simulink model "taskBasedBalancing"  (Simulink 9.0)
settings: Solver=FixedStepDiscrete  StartTime=0.0  StopTime=Config.t_end  FixedStep=Config.t_step  RelTol=1e-3  EnableMultiTasking=on
InitFcn:
  | cd(fileparts(which(bdroot)));
  | initTaskBasedBalancing;
StopFcn:
  | cd(fileparts(which(bdroot)));
  | stopTaskBasedBalancing;
undefined symbols (not defined in the file or in its folder): Config, DiscIntNeverNeededParam, Gains, ROBOT_DOF, Sat
libraries: WBToolboxLibrary x66
(part 2 of 2)

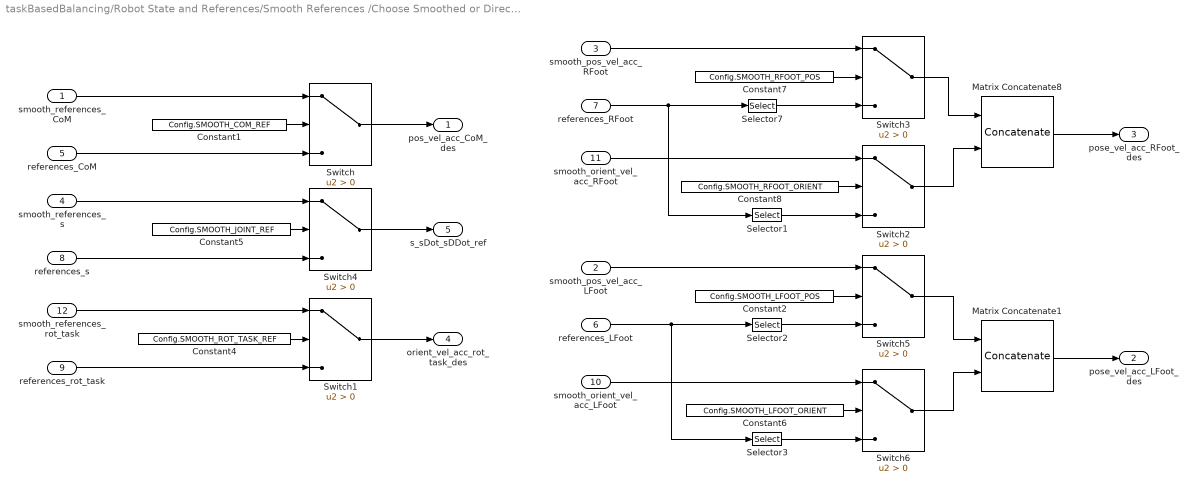
== system taskBasedBalancing/Robot State and References/Smooth References /Choose Smoothed or Direct References ==
  smooth_references_CoM : Inport
  smooth_pos_vel_acc_LFoot : Inport  Port=2
  smooth_pos_vel_acc_RFoot : Inport  Port=3
  smooth_references_s : Inport  Port=4
  references_CoM : Inport  Port=5
  references_LFoot : Inport  Port=6
  references_RFoot : Inport  Port=7
  references_s : Inport  Port=8
  references_rot_task : Inport  Port=9
  smooth_orient_vel_acc_LFoot : Inport  Port=10
  smooth_orient_vel_acc_RFoot : Inport  Port=11
  smooth_references_rot_task : Inport  Port=12
  Constant1 : Constant  Value=Config.SMOOTH_COM_REF
  Constant2 : Constant  Value=Config.SMOOTH_LFOOT_POS
  Constant4 : Constant  Value=Config.SMOOTH_ROT_TASK_REF
  Constant5 : Constant  Value=Config.SMOOTH_JOINT_REF
  Constant6 : Constant  Value=Config.SMOOTH_LFOOT_ORIENT
  Constant7 : Constant  Value=Config.SMOOTH_RFOOT_POS
  Constant8 : Constant  Value=Config.SMOOTH_RFOOT_ORIENT
  Matrix Concatenate1 : Concatenate  Mode=Multidimensional array
  Matrix Concatenate8 : Concatenate  Mode=Multidimensional array
  Selector1 : Selector  NumberOfDimensions=2  InputPortWidth=ROBOT_DOF  IndexOptions=Index vector (dialog),Index vector (dialog)  Indices=[4:6],[1:5]  OutputSizes=1,1
  Selector2 : Selector  NumberOfDimensions=2  InputPortWidth=ROBOT_DOF  IndexOptions=Index vector (dialog),Index vector (dialog)  Indices=[1:3],[1:5]  OutputSizes=1,1
  Selector3 : Selector  NumberOfDimensions=2  InputPortWidth=ROBOT_DOF  IndexOptions=Index vector (dialog),Index vector (dialog)  Indices=[4:6],[1:5]  OutputSizes=1,1
  Selector7 : Selector  NumberOfDimensions=2  InputPortWidth=ROBOT_DOF  IndexOptions=Index vector (dialog),Index vector (dialog)  Indices=[1:3],[1:5]  OutputSizes=1,1
  Switch{,1..6} (7 alike) : Switch  Criteria=u2 > Threshold
  pos_vel_acc_CoM_des : Outport
  pose_vel_acc_LFoot_des : Outport  Port=2
  pose_vel_acc_RFoot_des : Outport  Port=3
  orient_vel_acc_rot_task_des : Outport  Port=4
  s_sDot_sDDot_ref : Outport  Port=5
  wires:
  Constant1/1 -> Switch/2
  Switch/1 -> pos_vel_acc_CoM_des/1
  Constant5/1 -> Switch4/2
  Switch4/1 -> s_sDot_sDDot_ref/1
  references_CoM/1 -> Switch/3
  smooth_references_CoM/1 -> Switch/1
  smooth_references_s/1 -> Switch4/1
  references_s/1 -> Switch4/3
  smooth_references_rot_task/1 -> Switch1/1
  references_rot_task/1 -> Switch1/3
  Constant4/1 -> Switch1/2
  Switch1/1 -> orient_vel_acc_rot_task_des/1
  smooth_pos_vel_acc_RFoot/1 -> Switch3/1
  Constant7/1 -> Switch3/2
  references_RFoot/1 -> Selector1/1, Selector7/1
  Selector7/1 -> Switch3/3
  smooth_orient_vel_acc_RFoot/1 -> Switch2/1
  Constant8/1 -> Switch2/2
  Selector1/1 -> Switch2/3
  Switch3/1 -> Matrix Concatenate8/1
  Switch2/1 -> Matrix Concatenate8/2
  references_LFoot/1 -> Selector3/1, Selector2/1
  Matrix Concatenate8/1 -> pose_vel_acc_RFoot_des/1
  Constant6/1 -> Switch6/2
  Matrix Concatenate1/1 -> pose_vel_acc_LFoot_des/1
  Switch5/1 -> Matrix Concatenate1/1
  Switch6/1 -> Matrix Concatenate1/2
  Constant2/1 -> Switch5/2
  Selector2/1 -> Switch5/3
  smooth_pos_vel_acc_LFoot/1 -> Switch5/1
  smooth_orient_vel_acc_LFoot/1 -> Switch6/1
  Selector3/1 -> Switch6/3

== system taskBasedBalancing/Robot State and References/Smooth References /Smooth Reference Orientations ==
  w_R_LFoot_des : Inport
  w_R_RFoot_des : Inport  Port=2
  w_R_Rot_task_des : Inport  Port=3
  state : Inport  Port=4
  Compose Smoothed References : Subsystem
  Compute Smoothed Ref Orientations : Subsystem
  Constant{,1..5} (6 alike) : Constant  Value=zeros(3,1)
  smooth_orient_vel_acc_LFoot : Outport
  smooth_orient_vel_acc_RFoot : Outport  Port=2
  smooth_orient_vel_acc_Rot_task : Outport  Port=3
  wires:
  w_R_LFoot_des/1 -> Compute Smoothed Ref Orientations/1(w_R_LFoot_des)
  w_R_RFoot_des/1 -> Compute Smoothed Ref Orientations/2(w_R_RFoot_des)
  w_R_Rot_task_des/1 -> Compute Smoothed Ref Orientations/3(w_R_rot_task_des)
  Compute Smoothed Ref Orientations/3(w_R_LFoot) -> Compose Smoothed References/6(w_R_LFoot)
  Compute Smoothed Ref Orientations/2(w_R_RFoot) -> Compose Smoothed References/5(w_R_RFoot)
  Compute Smoothed Ref Orientations/1(w_R_rot_task) -> Compose Smoothed References/4(w_R_rot_task)
  Compose Smoothed References/1(orient_vel_acc_LFoot_des) -> smooth_orient_vel_acc_LFoot/1
  Compose Smoothed References/2(orient_vel_acc_RFoot_des) -> smooth_orient_vel_acc_RFoot/1
  Compose Smoothed References/3(orient_vel_acc_rot_task_des) -> smooth_orient_vel_acc_Rot_task/1
  state/1 -> Compute Smoothed Ref Orientations/4(state)
  Constant/1 -> Compose Smoothed References/1(omegaDot_LFoot)
  Constant1/1 -> Compose Smoothed References/2(omegaDot_RFoot)
  Constant2/1 -> Compose Smoothed References/3(omegaDot_rot_task)
  Constant5/1 -> Compose Smoothed References/9(omega_rot_task)
  Constant4/1 -> Compose Smoothed References/8(omega_RFoot)
  Constant3/1 -> Compose Smoothed References/7(omega_LFoot)

== system taskBasedBalancing/Robot State and References/Smooth References /Smooth Reference Positions ==
  pos_CoM_des : Inport
  pos_LFoot_des : Inport  Port=2
  pos_RFoot_des : Inport  Port=3
  s_des : Inport  Port=4
  state : Inport  Port=5
  Configure Settling Times : MATLAB Function  TreatAsAtomicUnit=on
  Matrix Concatenate1 : Concatenate  NumInputs=3  Mode=Multidimensional array  ConcatenateDimension=2
  Matrix Concatenate2 : Concatenate  NumInputs=4  Mode=Multidimensional array  ConcatenateDimension=2
  Matrix Concatenate3 : Concatenate  NumInputs=4  Mode=Multidimensional array  ConcatenateDimension=2
  Matrix Concatenate4 : Concatenate  NumInputs=3  Mode=Multidimensional array  ConcatenateDimension=2
  Minimum Jerk Trajectory Generator{,1..3} (4 alike) : WBToolboxLibrary/Utilities/Minimum Jerk Trajectory Generator  externalSettlingTime=on  settlingTime=3  sampleTime=Config.t_step  resetOnSettlingTime=off  firstDerivatives=on  secondDerivatives=on  explicitInitialValue=off
      settings: SourceProductName=Whole Body Toolbox
  Settling time1 : Constant  Value=zeros(3,2)
  smooth_references_CoM : Outport
  smooth_pos_vel_acc_LFoot : Outport  Port=2
  smooth_pos_vel_acc_RFoot : Outport  Port=3
  smooth_references_s : Outport  Port=4
  wires:
  Minimum Jerk Trajectory Generator2/2 -> Matrix Concatenate3/2
  pos_LFoot_des/1 -> Minimum Jerk Trajectory Generator2/1
  pos_RFoot_des/1 -> Minimum Jerk Trajectory Generator3/1
  Minimum Jerk Trajectory Generator2/3 -> Matrix Concatenate3/3
  Minimum Jerk Trajectory Generator2/1 -> Matrix Concatenate3/1
  Minimum Jerk Trajectory Generator1/3 -> Matrix Concatenate1/3
  Matrix Concatenate1/1 -> smooth_references_s/1
  Matrix Concatenate4/1 -> smooth_references_CoM/1
  Minimum Jerk Trajectory Generator1/1 -> Matrix Concatenate1/1
  pos_CoM_des/1 -> Minimum Jerk Trajectory Generator/1
  Minimum Jerk Trajectory Generator/3 -> Matrix Concatenate4/3
  Minimum Jerk Trajectory Generator/2 -> Matrix Concatenate4/2
  Minimum Jerk Trajectory Generator1/2 -> Matrix Concatenate1/2
  Minimum Jerk Trajectory Generator3/3 -> Matrix Concatenate2/3
  Matrix Concatenate3/1 -> smooth_pos_vel_acc_LFoot/1
  Matrix Concatenate2/1 -> smooth_pos_vel_acc_RFoot/1
  Minimum Jerk Trajectory Generator/1 -> Matrix Concatenate4/1
  Minimum Jerk Trajectory Generator3/2 -> Matrix Concatenate2/2
  s_des/1 -> Minimum Jerk Trajectory Generator1/1
  Settling time1/1 -> Matrix Concatenate2/4, Matrix Concatenate3/4
  Minimum Jerk Trajectory Generator3/1 -> Matrix Concatenate2/1
  state/1 -> Configure Settling Times/1(state)
  Configure Settling Times/1(smoothingTime_CoM) -> Minimum Jerk Trajectory Generator/2
  Configure Settling Times/2(smoothingTime_joints) -> Minimum Jerk Trajectory Generator1/2
  Configure Settling Times/3(smoothingTime_LFoot) -> Minimum Jerk Trajectory Generator2/2
  Configure Settling Times/4(smoothingTime_RFoot) -> Minimum Jerk Trajectory Generator3/2

== system taskBasedBalancing/Robot State and References/State Machine/Compute Transformation Matrices ==
  s : Inport
  IMU port : Inport  Port=2
  Constant : Constant  Value=Config.LEFT_FOOT_IN_CONTACT
  Constant6 : Constant  Value=eye(4)
  "Inv\\*  " : Product  Inputs=/  Multiplication=Matrix(*)
  LFoot to base link transform : Subsystem
  LFoot to world transform (fixed base) : WBToolboxLibrary/wholeBodyModel/Kinematics/Forward Kinematics  frameName=Frames.LEFT_FOOT
      settings: SourceProductName=Whole Body Toolbox
  RFoot to base link transform : Subsystem
  RFoot to world transform (fixed base) : WBToolboxLibrary/wholeBodyModel/Kinematics/Forward Kinematics  frameName=Frames.RIGHT_FOOT
      settings: SourceProductName=Whole Body Toolbox
  Switch : Switch  Criteria=u2 > Threshold
  w_H_b_initial : Outport
  b_H_LFoot : Outport  Port=2
  b_H_RFoot : Outport  Port=3
  wires:
  s/1 -> RFoot to world transform (fixed base)/2, LFoot to world transform (fixed base)/2, RFoot to base link transform/1(s), LFoot to base link transform/1(s)
  RFoot to base link transform/1(b_H_link_corrected) -> Switch/3, b_H_RFoot/1
  LFoot to world transform (fixed base)/1 -> LFoot to base link transform/3(b_H_link)
  IMU port/1 -> RFoot to base link transform/2(inertial), LFoot to base link transform/2(inertial)
  Constant6/1 -> LFoot to world transform (fixed base)/1, RFoot to world transform (fixed base)/1
  RFoot to world transform (fixed base)/1 -> RFoot to base link transform/3(b_H_link)
  LFoot to base link transform/1(b_H_link_corrected) -> Switch/1, b_H_LFoot/1
  Switch/1 -> "Inv\\*  "/1
  Constant/1 -> Switch/2
  "Inv\\*  "/1 -> w_H_b_initial/1

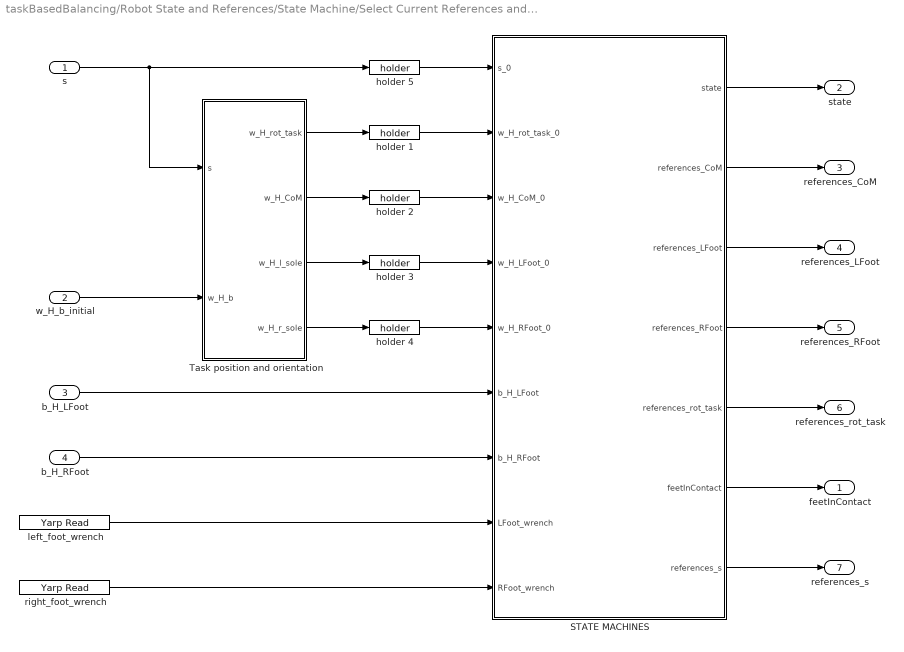
== system taskBasedBalancing/Robot State and References/State Machine/Select Current References and Estimate w_H_b ==
  s : Inport
  w_H_b_initial : Inport  Port=2
  b_H_LFoot : Inport  Port=3
  b_H_RFoot : Inport  Port=4
  STATE MACHINES : MATLAB Function  TreatAsAtomicUnit=on
  Task position and orientation : Subsystem
  holder {1..5} (5 alike) : WBToolboxLibrary/Utilities/holder 
      settings: SourceProductName=Whole Body Toolbox
  left_foot_wrench : WBToolboxLibrary/Utilities/Yarp Read  portName=Ports.LEFT_FOOT_EXT_WRENCH  signalSize=6  timeout=0.5  blocking=off  timestamp=off  autoconnect=on  errorOnConnection=on
      settings: SourceProductName=Whole Body Toolbox
  right_foot_wrench : WBToolboxLibrary/Utilities/Yarp Read  portName=Ports.RIGHT_FOOT_EXT_WRENCH  signalSize=6  timeout=0.5  blocking=off  timestamp=off  autoconnect=on  errorOnConnection=on
      settings: SourceProductName=Whole Body Toolbox
  feetInContact : Outport
  state : Outport  Port=2
  references_CoM : Outport  Port=3
  references_LFoot : Outport  Port=4
  references_RFoot : Outport  Port=5
  references_rot_task : Outport  Port=6
  references_s : Outport  Port=7
  wires:
  s/1 -> Task position and orientation/1(s), holder 5/1
  w_H_b_initial/1 -> Task position and orientation/2(w_H_b)
  holder 5/1 -> STATE MACHINES/1(s_0)
  Task position and orientation/1(w_H_rot_task) -> holder 1/1
  holder 1/1 -> STATE MACHINES/2(w_H_rot_task_0)
  b_H_RFoot/1 -> STATE MACHINES/7(b_H_RFoot)
  b_H_LFoot/1 -> STATE MACHINES/6(b_H_LFoot)
  left_foot_wrench/1 -> STATE MACHINES/8(LFoot_wrench)
  right_foot_wrench/1 -> STATE MACHINES/9(RFoot_wrench)
  STATE MACHINES/1(state) -> state/1
  STATE MACHINES/2(references_CoM) -> references_CoM/1
  STATE MACHINES/3(references_LFoot) -> references_LFoot/1
  STATE MACHINES/4(references_RFoot) -> references_RFoot/1
  STATE MACHINES/5(references_rot_task) -> references_rot_task/1
  STATE MACHINES/6(feetInContact) -> feetInContact/1
  STATE MACHINES/7(references_s) -> references_s/1
  Task position and orientation/4(w_H_r_sole) -> holder 4/1
  Task position and orientation/3(w_H_l_sole) -> holder 3/1
  Task position and orientation/2(w_H_CoM) -> holder 2/1
  holder 4/1 -> STATE MACHINES/5(w_H_RFoot_0)
  holder 3/1 -> STATE MACHINES/4(w_H_LFoot_0)
  holder 2/1 -> STATE MACHINES/3(w_H_CoM_0)

== system taskBasedBalancing/Robot State and References/State Machine/emergency stop: joint limits ==
  s   EMERGENCY STOP : Inport
  Enable : EnablePort
  Assertion : Assertion
  Get Limits : WBToolboxLibrary/wholeBodyStates/Get Limits  limitsSource=ControlBoard  limitsType=Position
      settings: SourceProductName=Whole Body Toolbox
  MATLAB Function : MATLAB Function  TreatAsAtomicUnit=on
  index1 : Constant  Value=0.01  VectorParams1D=off
  wires:
  Get Limits/1 -> MATLAB Function/1(umin)
  Get Limits/2 -> MATLAB Function/2(umax)
  index1/1 -> MATLAB Function/4(tol)
  s   EMERGENCY STOP/1 -> MATLAB Function/3(u)
  MATLAB Function/1(inRange) -> Assertion/1

== system taskBasedBalancing/Visualization/Visualize Smoothing (orientation)/Rotation Error Left Foot ==
  w_R_LFoot : Inport
  w_R_LFoot_des : Inport  Port=2
  Permute Dimensions2 : PermuteDimensions
  Product2 : Product  Multiplication=Matrix(*)
  Rot error using roll-pitch-yaw : MATLAB Function  TreatAsAtomicUnit=on
  rollPitchYaw : Outport
  wires:
  w_R_LFoot_des/1 -> Product2/2
  w_R_LFoot/1 -> Permute Dimensions2/1
  Permute Dimensions2/1 -> Product2/1
  Rot error using roll-pitch-yaw/1(rollPitchYaw) -> rollPitchYaw/1
  Product2/1 -> Rot error using roll-pitch-yaw/1(R_0)

== system taskBasedBalancing/Visualization/Visualize Smoothing (orientation)/Rotation Error Right Foot ==
  w_R_RFoot : Inport
  w_R_RFoot_des : Inport  Port=2
  Permute Dimensions2 : PermuteDimensions
  Product2 : Product  Multiplication=Matrix(*)
  Rot error using roll-pitch-yaw : MATLAB Function  TreatAsAtomicUnit=on
  rollPitchYaw : Outport
  wires:
  w_R_RFoot_des/1 -> Product2/2
  w_R_RFoot/1 -> Permute Dimensions2/1
  Permute Dimensions2/1 -> Product2/1
  Rot error using roll-pitch-yaw/1(rollPitchYaw) -> rollPitchYaw/1
  Product2/1 -> Rot error using roll-pitch-yaw/1(R_0)

== system taskBasedBalancing/Visualization/Visualize Smoothing (orientation)/Rotation Error Rot Task ==
  w_R_rot_task : Inport
  w_R_rot_task_des : Inport  Port=2
  Permute Dimensions2 : PermuteDimensions
  Product2 : Product  Multiplication=Matrix(*)
  Rot error using roll-pitch-yaw : MATLAB Function  TreatAsAtomicUnit=on
  rollPitchYaw : Outport
  wires:
  w_R_rot_task_des/1 -> Product2/2
  w_R_rot_task/1 -> Permute Dimensions2/1
  Permute Dimensions2/1 -> Product2/1
  Rot error using roll-pitch-yaw/1(rollPitchYaw) -> rollPitchYaw/1
  Product2/1 -> Rot error using roll-pitch-yaw/1(R_0)

== system taskBasedBalancing/Robot State and References/Smooth References /Smooth Reference Orientations/Compose Smoothed References ==
  omegaDot_LFoot : Inport
  omegaDot_RFoot : Inport  Port=2
  omegaDot_rot_task : Inport  Port=3
  w_R_rot_task : Inport  Port=4
  w_R_RFoot : Inport  Port=5
  w_R_LFoot : Inport  Port=6
  omega_LFoot : Inport  Port=7
  omega_RFoot : Inport  Port=8
  omega_rot_task : Inport  Port=9
  Matrix Concatenate1 : Concatenate  NumInputs=3  Mode=Multidimensional array  ConcatenateDimension=2
  Matrix Concatenate2 : Concatenate  NumInputs=3  Mode=Multidimensional array  ConcatenateDimension=2
  Matrix Concatenate6 : Concatenate  NumInputs=3  Mode=Multidimensional array  ConcatenateDimension=2
  orient_vel_acc_LFoot_des : Outport
  orient_vel_acc_RFoot_des : Outport  Port=2
  orient_vel_acc_rot_task_des : Outport  Port=3
  wires:
  w_R_LFoot/1 -> Matrix Concatenate6/1
  Matrix Concatenate6/1 -> orient_vel_acc_LFoot_des/1
  Matrix Concatenate2/1 -> orient_vel_acc_rot_task_des/1
  Matrix Concatenate1/1 -> orient_vel_acc_RFoot_des/1
  omega_LFoot/1 -> Matrix Concatenate6/2
  omega_RFoot/1 -> Matrix Concatenate1/2
  w_R_RFoot/1 -> Matrix Concatenate1/1
  omega_rot_task/1 -> Matrix Concatenate2/2
  w_R_rot_task/1 -> Matrix Concatenate2/1
  omegaDot_LFoot/1 -> Matrix Concatenate6/3
  omegaDot_RFoot/1 -> Matrix Concatenate1/3
  omegaDot_rot_task/1 -> Matrix Concatenate2/3

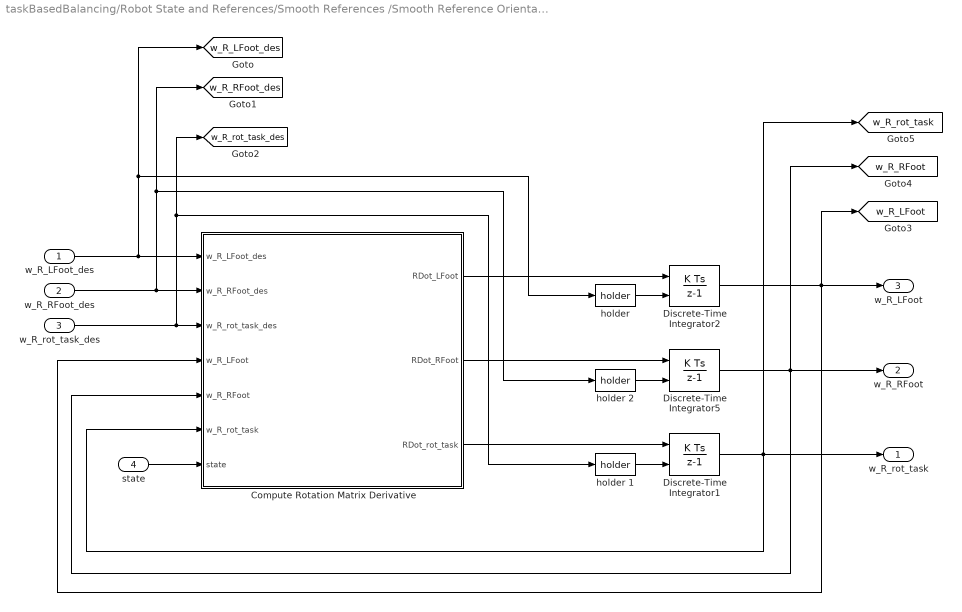
== system taskBasedBalancing/Robot State and References/Smooth References /Smooth Reference Orientations/Compute Smoothed Ref Orientations ==
  w_R_LFoot_des : Inport
  w_R_RFoot_des : Inport  Port=2
  w_R_rot_task_des : Inport  Port=3
  state : Inport  Port=4
  Compute Rotation Matrix Derivative : MATLAB Function  TreatAsAtomicUnit=on
  Discrete-Time Integrator1 : DiscreteIntegrator  InitialConditionSource=external  InitialCondition=zeros(3,1)  InitialConditionSetting=State (most efficient)  SampleTime=Config.t_step  ICPrevOutput=DiscIntNeverNeededParam  ICPrevScaledInput=DiscIntNeverNeededParam
  Discrete-Time Integrator2 : DiscreteIntegrator  InitialConditionSource=external  InitialCondition=zeros(3,1)  InitialConditionSetting=State (most efficient)  SampleTime=Config.t_step  ICPrevOutput=DiscIntNeverNeededParam  ICPrevScaledInput=DiscIntNeverNeededParam
  Discrete-Time Integrator5 : DiscreteIntegrator  InitialConditionSource=external  InitialCondition=zeros(3,1)  InitialConditionSetting=State (most efficient)  SampleTime=Config.t_step  ICPrevOutput=DiscIntNeverNeededParam  ICPrevScaledInput=DiscIntNeverNeededParam
  "holder " : WBToolboxLibrary/Utilities/holder 
      settings: SourceProductName=Whole Body Toolbox
  holder 1 : WBToolboxLibrary/Utilities/holder 
      settings: SourceProductName=Whole Body Toolbox
  holder 2 : WBToolboxLibrary/Utilities/holder 
      settings: SourceProductName=Whole Body Toolbox
  w_R_rot_task : Outport
  w_R_RFoot : Outport  Port=2
  w_R_LFoot : Outport  Port=3
  tag scope: w_R_LFoot=global, w_R_LFoot_des=global, w_R_RFoot=global, w_R_RFoot_des=global, w_R_rot_task=global, w_R_rot_task_des=global
  wires:
  "holder "/1 -> Discrete-Time Integrator2/2
  holder 2/1 -> Discrete-Time Integrator5/2
  holder 1/1 -> Discrete-Time Integrator1/2
  Compute Rotation Matrix Derivative/1(RDot_LFoot) -> Discrete-Time Integrator2/1
  Compute Rotation Matrix Derivative/2(RDot_RFoot) -> Discrete-Time Integrator5/1
  Compute Rotation Matrix Derivative/3(RDot_rot_task) -> Discrete-Time Integrator1/1
  Discrete-Time Integrator5/1 -> w_R_RFoot/1, [w_R_RFoot], Compute Rotation Matrix Derivative/5(w_R_RFoot)
  Discrete-Time Integrator1/1 -> [w_R_rot_task], w_R_rot_task/1, Compute Rotation Matrix Derivative/6(w_R_rot_task)
  Discrete-Time Integrator2/1 -> [w_R_LFoot], w_R_LFoot/1, Compute Rotation Matrix Derivative/4(w_R_LFoot)
  w_R_LFoot_des/1 -> Compute Rotation Matrix Derivative/1(w_R_LFoot_des), [w_R_LFoot_des], "holder "/1
  w_R_RFoot_des/1 -> Compute Rotation Matrix Derivative/2(w_R_RFoot_des), [w_R_RFoot_des], holder 2/1
  w_R_rot_task_des/1 -> Compute Rotation Matrix Derivative/3(w_R_rot_task_des), holder 1/1, [w_R_rot_task_des]
  state/1 -> Compute Rotation Matrix Derivative/7(state)

== system taskBasedBalancing/Robot State and References/State Machine/Compute Transformation Matrices/LFoot to base link transform ==
  s : Inport
  inertial : Inport  Port=2
  b_H_link : Inport  Port=3
  Constant6 : Constant  Value=eye(4)
  Fixed base to imu transform : WBToolboxLibrary/wholeBodyModel/Kinematics/Forward Kinematics  frameName=Frames.IMU
      settings: SourceProductName=Whole Body Toolbox
  Inv\* : Product  Inputs=/*  Multiplication=Matrix(*)
  "Inv\\*  " : Product  Inputs=/  Multiplication=Matrix(*)
  Inv\*  1 : Product  Inputs=/  Multiplication=Matrix(*)
  Neck Position : WBToolboxLibrary/Utilities/Yarp Read  portName=Ports.NECK_POS  signalSize=6  timeout=0.5  blocking=off  timestamp=off  autoconnect=on  errorOnConnection=off
      settings: SourceProductName=Whole Body Toolbox
  Switch6 : Switch  Criteria=u2 > Threshold
  USE_IMU4EST_BASE : Constant  Value=Config.USE_IMU4EST_BASE
  fromImuToHomogeousTransformFCN : MATLAB Function  TreatAsAtomicUnit=on
  holder 1 : WBToolboxLibrary/Utilities/holder 
      settings: SourceProductName=Whole Body Toolbox
  holder 2 : WBToolboxLibrary/Utilities/holder 
      settings: SourceProductName=Whole Body Toolbox
  neck transform : Subsystem
  b_H_link_corrected : Outport
  wires:
  Switch6/1 -> b_H_link_corrected/1
  "Inv\\*  "/1 -> fromImuToHomogeousTransformFCN/3(link_H_base)  "link_H_b"
  USE_IMU4EST_BASE/1 -> Switch6/2
  Inv\*/1 -> fromImuToHomogeousTransformFCN/1(imu_H_link), holder 1/1  "imu_H_link"
  holder 2/1 -> fromImuToHomogeousTransformFCN/4(inertial_0)
  Fixed base to imu transform/1 -> Inv\*/1
  holder 1/1 -> fromImuToHomogeousTransformFCN/2(imu_H_link_0)
  s/1 -> Fixed base to imu transform/2
  fromImuToHomogeousTransformFCN/1(w_H_b) -> Inv\*  1/1
  inertial/1 -> holder 2/1, fromImuToHomogeousTransformFCN/5(inertial)
  Neck Position/1 -> neck transform/1(neck port)
  neck transform/1(neck position) -> fromImuToHomogeousTransformFCN/6(neck_pos)
  b_H_link/1 -> Switch6/3, "Inv\\*  "/1, Inv\*/2
  Constant6/1 -> Fixed base to imu transform/1
  Inv\*  1/1 -> Switch6/1

== system taskBasedBalancing/Robot State and References/State Machine/Compute Transformation Matrices/RFoot to base link transform ==
  s : Inport
  inertial : Inport  Port=2
  b_H_link : Inport  Port=3
  Constant6 : Constant  Value=eye(4)
  Fixed base to imu transform : WBToolboxLibrary/wholeBodyModel/Kinematics/Forward Kinematics  frameName=Frames.IMU
      settings: SourceProductName=Whole Body Toolbox
  Inv\* : Product  Inputs=/*  Multiplication=Matrix(*)
  "Inv\\*  " : Product  Inputs=/  Multiplication=Matrix(*)
  Inv\*  1 : Product  Inputs=/  Multiplication=Matrix(*)
  Neck Position : WBToolboxLibrary/Utilities/Yarp Read  portName=Ports.NECK_POS  signalSize=6  timeout=0.5  blocking=off  timestamp=off  autoconnect=on  errorOnConnection=off
      settings: SourceProductName=Whole Body Toolbox
  Switch6 : Switch  Criteria=u2 > Threshold
  USE_IMU4EST_BASE : Constant  Value=Config.USE_IMU4EST_BASE
  fromImuToHomogeousTransformFCN : MATLAB Function  TreatAsAtomicUnit=on
  holder 1 : WBToolboxLibrary/Utilities/holder 
      settings: SourceProductName=Whole Body Toolbox
  holder 2 : WBToolboxLibrary/Utilities/holder 
      settings: SourceProductName=Whole Body Toolbox
  neck transform : Subsystem
  b_H_link_corrected : Outport
  wires:
  Switch6/1 -> b_H_link_corrected/1
  "Inv\\*  "/1 -> fromImuToHomogeousTransformFCN/3(link_H_base)  "link_H_b"
  USE_IMU4EST_BASE/1 -> Switch6/2
  Inv\*/1 -> fromImuToHomogeousTransformFCN/1(imu_H_link), holder 1/1  "imu_H_link"
  holder 2/1 -> fromImuToHomogeousTransformFCN/4(inertial_0)
  Fixed base to imu transform/1 -> Inv\*/1
  holder 1/1 -> fromImuToHomogeousTransformFCN/2(imu_H_link_0)
  s/1 -> Fixed base to imu transform/2
  fromImuToHomogeousTransformFCN/1(w_H_b) -> Inv\*  1/1
  inertial/1 -> holder 2/1, fromImuToHomogeousTransformFCN/5(inertial)
  Neck Position/1 -> neck transform/1(neck port)
  neck transform/1(neck position) -> fromImuToHomogeousTransformFCN/6(neck_pos)
  b_H_link/1 -> Switch6/3, "Inv\\*  "/1, Inv\*/2
  Constant6/1 -> Fixed base to imu transform/1
  Inv\*  1/1 -> Switch6/1

== system taskBasedBalancing/Robot State and References/State Machine/Select Current References and Estimate w_H_b/Task position and orientation ==
  s : Inport
  w_H_b : Inport  Port=2
  CoM : WBToolboxLibrary/wholeBodyModel/Kinematics/Forward Kinematics  frameName=Frames.COM
      settings: SourceProductName=Whole Body Toolbox
  LFoot : WBToolboxLibrary/wholeBodyModel/Kinematics/Forward Kinematics  frameName=Frames.LEFT_FOOT
      settings: SourceProductName=Whole Body Toolbox
  RFoot : WBToolboxLibrary/wholeBodyModel/Kinematics/Forward Kinematics  frameName=Frames.RIGHT_FOOT
      settings: SourceProductName=Whole Body Toolbox
  rotational task : WBToolboxLibrary/wholeBodyModel/Kinematics/Forward Kinematics  frameName=Frames.ROT_TASK_LINK
      settings: SourceProductName=Whole Body Toolbox
  w_H_rot_task : Outport
  w_H_CoM : Outport  Port=2
  w_H_l_sole : Outport  Port=3
  w_H_r_sole : Outport  Port=4
  wires:
  s/1 -> rotational task/2, RFoot/2, LFoot/2, CoM/2
  w_H_b/1 -> rotational task/1, CoM/1, LFoot/1, RFoot/1
  CoM/1 -> w_H_CoM/1
  LFoot/1 -> w_H_l_sole/1
  RFoot/1 -> w_H_r_sole/1
  rotational task/1 -> w_H_rot_task/1

== system taskBasedBalancing/Robot State and References/State Machine/Compute Transformation Matrices/LFoot to base link transform/neck transform ==
  neck port : Inport
  Constant : Constant  Value=zeros(3,1)
  Gain : Gain  Gain=pi/180
  Selector1 : Selector  InputPortWidth=6  IndexOptions=Index vector (dialog)  Indices=[1:3]  OutputSizes=1
  Switch : Switch  Criteria=u2 > Threshold
  USE_IMU4EST_BASE1 : Constant  Value=Config.CORRECT_IMU_WITH_NECK_POS
  neck position : Outport
  wires:
  neck port/1 -> Gain/1
  USE_IMU4EST_BASE1/1 -> Switch/2
  Switch/1 -> neck position/1
  Gain/1 -> Selector1/1
  Constant/1 -> Switch/3
  Selector1/1 -> Switch/1  "neck pos"

== system taskBasedBalancing/Robot State and References/State Machine/Compute Transformation Matrices/RFoot to base link transform/neck transform ==
  neck port : Inport
  Constant : Constant  Value=zeros(3,1)
  Gain : Gain  Gain=pi/180
  Selector1 : Selector  InputPortWidth=6  IndexOptions=Index vector (dialog)  Indices=[1:3]  OutputSizes=1
  Switch : Switch  Criteria=u2 > Threshold
  USE_IMU4EST_BASE1 : Constant  Value=Config.CORRECT_IMU_WITH_NECK_POS
  neck position : Outport
  wires:
  neck port/1 -> Gain/1
  USE_IMU4EST_BASE1/1 -> Switch/2
  Switch/1 -> neck position/1
  Gain/1 -> Selector1/1
  Constant/1 -> Switch/3
  Selector1/1 -> Switch/1  "neck pos"

== matlab function Initial Conditions/compute state velocity/Compute Base Velocity ==
  data: J_LeftFoot input double; J_RightFoot input double; feetInContact input double; nu_b output double; sDot input double; Sat parameter double
function nu_b = computeBaseVelocityFCN(J_LeftFoot, J_RightFoot, feetInContact, sDot, Sat)

    nu_b = computeBaseVelocity(J_LeftFoot, J_RightFoot, feetInContact, sDot, Sat);
end

== matlab function Inverse Kinematics/Compute tasks accelerations ==
  data: pos_vel_acc_CoM_des input double; acc_task_star output double; pose_vel_acc_LFoot_des input double; pose_vel_acc_RFoot_des input double; orient_vel_acc_rot_task_des input double; pos_vel_CoM input double; pose_vel_LFoot input double; pose_vel_RFoot input double; orient_vel_rot_task input double; Kp_Kd_CoM input double; Kp_Kd_LFoot input double; Kp_Kd_RFoot input double; Kp_Kd_rot_task input double; useFeetPIDs input double; Sat parameter double
function acc_task_star = setTasksAccelerationsFCN(pos_vel_acc_CoM_des,pose_vel_acc_LFoot_des,pose_vel_acc_RFoot_des,orient_vel_acc_rot_task_des, ...
                                                  pos_vel_CoM, pose_vel_LFoot, pose_vel_RFoot, orient_vel_rot_task, ...
                                                  Kp_Kd_CoM, Kp_Kd_LFoot, Kp_Kd_RFoot, Kp_Kd_rot_task, useFeetPIDs, Sat) 

    acc_task_star = setTasksAccelerations(pos_vel_acc_CoM_des,pose_vel_acc_LFoot_des,pose_vel_acc_RFoot_des,orient_vel_acc_rot_task_des, ...
                                          pos_vel_CoM, pose_vel_LFoot, pose_vel_RFoot, orient_vel_rot_task, ...
                                          Kp_Kd_CoM, Kp_Kd_LFoot, Kp_Kd_RFoot, Kp_Kd_rot_task, useFeetPIDs, Sat);  
end

== matlab function Inverse Kinematics/ComputeTasksPoseAndVelocity/Compose Task Pose and Velocity ==
  data: vel_CoM input double; vel_LFoot input double; vel_RFoot input double; vel_rot_task input double; pos_vel_CoM output double; pose_vel_LFoot output double; pose_vel_RFoot output double; orient_vel_rot_task output double; w_H_CoM input double; w_H_l_sole input double; w_H_r_sole input double; w_H_rot_task input double
function [pos_vel_CoM, pose_vel_LFoot, pose_vel_RFoot, orient_vel_rot_task] = ...
             composeTaskPoseAndVelocityFCN(vel_CoM, vel_LFoot, vel_RFoot, vel_rot_task, ...
                                           w_H_CoM, w_H_l_sole, w_H_r_sole, w_H_rot_task)
                                                                                                                              
    [pos_vel_CoM, pose_vel_LFoot, pose_vel_RFoot, orient_vel_rot_task] = ...
       composeTaskPoseAndVelocity(vel_CoM, vel_LFoot, vel_RFoot, vel_rot_task, ...
                                  w_H_CoM, w_H_l_sole, w_H_r_sole, w_H_rot_task);
                              
end

== matlab function Inverse Kinematics/QP-Based Inverse Kinematics/Compute QP Hessian, gradient and constraints  ==
  data: s input double; nu input double; s_sDot_sDDot_ref input double; Hessian output double; impedances input double; dampings input double; J input double; JDot_nu input double; acc_task_star input double; gradient output double; ConstraintMatrix output double; biasVectorConstraint output double
function [Hessian, gradient, ConstraintMatrix, biasVectorConstraint] = ...
             computeQPHessianAndConstraintsFCN(s, nu, s_sDot_sDDot_ref, impedances, dampings, J, JDot_nu, acc_task_star)
    
    [Hessian, gradient, ConstraintMatrix, biasVectorConstraint] = ...
        computeQPHessianAndConstraints(s, nu, s_sDot_sDDot_ref, impedances, dampings, J, JDot_nu, acc_task_star);
end

== matlab function Robot State and References/Gain Scheduling/Gain Scheduling Function ==
  data: state input double; Kp_CoM output double; Kd_CoM output double; Kp_LFoot output double; Kd_LFoot output double; Kp_RFoot output double; Kd_RFoot output double; Kp_rot_task output double; Kd_rot_task output double; impedances output double; dampings output double; Gains parameter double; smoothingTimeGains output double; Config parameter double
function [Kp_CoM, Kd_CoM, Kp_LFoot, Kd_LFoot, Kp_RFoot, Kd_RFoot, Kp_rot_task, Kd_rot_task, impedances, dampings, smoothingTimeGains] = ...
             gainSchedulingFCN(state,Gains,Config)

    [Kp_CoM, Kd_CoM, Kp_LFoot, Kd_LFoot, Kp_RFoot, Kd_RFoot, Kp_rot_task, Kd_rot_task, impedances, dampings, smoothingTimeGains] = ...
        gainScheduling(state,Gains,Config);
end

== matlab function Robot State and References/State Machine/Select Current References and Estimate w_H_b/STATE MACHINES ==
  data: s_0 input double; w_H_rot_task_0 input double; w_H_CoM_0 input double; w_H_LFoot_0 input double; w_H_RFoot_0 input double; b_H_LFoot input double; b_H_RFoot input double; LFoot_wrench input double; RFoot_wrench input double; state output double; references_CoM output double; references_LFoot output double; references_RFoot output double; references_rot_task output double; feetInContact output double; references_s output double; Config parameter double; Sat parameter double
function [state, references_CoM, references_LFoot, references_RFoot, references_rot_task, feetInContact, references_s] = stateMachineBalancingFCN ...
             (s_0, w_H_rot_task_0, w_H_CoM_0, w_H_LFoot_0, w_H_RFoot_0, b_H_LFoot, b_H_RFoot, LFoot_wrench, RFoot_wrench, Config, Sat)
        
       % Position control balancing state machine
       [state, references_CoM, references_LFoot, references_RFoot, references_rot_task, feetInContact, references_s] = stateMachineBalancing ...
             (s_0, w_H_rot_task_0, w_H_CoM_0, w_H_LFoot_0, w_H_RFoot_0, b_H_LFoot, b_H_RFoot, LFoot_wrench, RFoot_wrench, Config, Sat);
        
end

== matlab function Robot State and References/Smooth References /Smooth Reference Orientations/Compute Smoothed Ref Orientations/Compute Rotation Matrix Derivative ==
  data: RDot_LFoot output double; RDot_RFoot output double; RDot_rot_task output double; w_R_LFoot_des input double; w_R_RFoot_des input double; w_R_rot_task_des input double; w_R_LFoot input double; w_R_RFoot input double; w_R_rot_task input double; state input double; Config parameter double
function [RDot_LFoot, RDot_RFoot, RDot_rot_task] = rotationDerivativeFromAngVelFCN(w_R_LFoot_des, w_R_RFoot_des, w_R_rot_task_des, ... 
                                                                                   w_R_LFoot, w_R_RFoot, w_R_rot_task, state, Config)
      
                                                                                                                                                         
    % Compute the input angular velocity (expressed in world frame)
    
    % Left foot
    w_omegaLFoot_des     = zeros(3,1);
    Kp_LFoot             = Config.LFoot_Kp_smoothing(state);
    w_omegaLFoot         = rotationalPID_velocity(w_R_LFoot,w_R_LFoot_des,w_omegaLFoot_des,Kp_LFoot);
    
    % Right foot
    w_omegaRFoot_des     = zeros(3,1);
    Kp_RFoot             = Config.RFoot_Kp_smoothing(state);
    w_omegaRFoot         = rotationalPID_velocity(w_R_RFoot,w_R_RFoot_des,w_omegaRFoot_des,Kp_RFoot);
    
    % Rot task
    w_omega_rot_task_des = zeros(3,1);
    Kp_rot_task          = Config.rot_task_Kp_smoothing(state);
    w_omega_rot_task     = rotationalPID_velocity(w_R_rot_task,w_R_rot_task_des,w_omega_rot_task_des,Kp_rot_task);
                                    
    % Compute the rotation matrix derivative given the angular velocity
    RDot_LFoot           = rotationDerivativeFromAngVel(w_omegaLFoot, w_R_LFoot);
    RDot_RFoot           = rotationDerivativeFromAngVel(w_omegaRFoot, w_R_RFoot);
    RDot_rot_task        = rotationDerivativeFromAngVel(w_omega_rot_task, w_R_rot_task);      
end

== matlab function Robot State and References/State Machine/Compute Transformation Matrices/RFoot to base link transform/fromImuToHomogeousTransformFCN ==
  data: imu_H_link input double; imu_H_link_0 input double; link_H_base input double; inertial_0 input double; inertial input double; neck_pos input double; w_H_b output double; Config parameter double
function w_H_b = worldToBaseTransformWithIMUFCN(imu_H_link,imu_H_link_0,link_H_base,inertial_0,inertial,neck_pos,Config)

    w_H_b = worldToBaseTransformWithIMU(imu_H_link,imu_H_link_0,link_H_base,inertial_0,inertial,neck_pos,Config);

end

== matlab function Inverse Kinematics/QP-Based Inverse Kinematics/inverse kinematics integration/Rewrite Base Pose as transformation matrix ==
  data: pose_b input double; w_H_b output double
function  w_H_b = fromPosQuatToTransfMatrFCN(pose_b) 

    % converts the base pose from a position + quaternion representation 
    % to a tranformation matrix
    w_H_b = fromPosQuatToTransfMatr(pose_b);
end

== matlab function Inverse Kinematics/QP-Based Inverse Kinematics/inverse kinematics integration/Compute Base Pose Derivative ==
  data: pose_b input double; nu_b input double; pose_bDot output double
function pose_bDot = basePoseDerivativeFCN(pose_b,nu_b)

    % time derivative of the floating base pose
    pose_bDot = basePoseDerivative(nu_b, pose_b);
end

== matlab function Robot State and References/Smooth References /Smooth Reference Positions/Configure Settling Times ==
  data: state input double; Config parameter double; smoothingTime_CoM output double; smoothingTime_joints output double; smoothingTime_LFoot output double; smoothingTime_RFoot output double
function [smoothingTime_CoM, smoothingTime_joints, smoothingTime_LFoot, smoothingTime_RFoot] = setSmoothingTimesFCN(state,Config)

    [smoothingTime_CoM, smoothingTime_LFoot, smoothingTime_RFoot, smoothingTime_joints] = setSmoothingTimes(state,Config);

end

== matlab function Inverse Kinematics/QP-Based Inverse Kinematics/inverse kinematics integration/Rewrite Base Pose as pos+quat ==
  data: w_H_b_0 input double; pose_b_0 output double
function pose_b_0 = fromTransfMatrixToPosQuatFCN(w_H_b_0)

    % converts the floating base pose expressed in terms of transformation
    % matrix into position + quaternion representation 
    pose_b_0 = fromTransfMatrixToPosQuat(w_H_b_0);

end

== matlab function Robot State and References/State Machine/emergency stop: joint limits/MATLAB Function ==
  data: umin input double; umax input double; u input double; inRange output double; tol input double
function inRange = checkRangeFCN(umin, umax, u, tol)

     inRange = checkRange(umin, umax, u, tol);
end

== matlab function Visualization/Visualize Smoothing (orientation)/Rotation Error Left Foot/Rot error using roll-pitch-yaw ==
  data: R_0 input double; rollPitchYaw output double
function rollPitchYaw = rollPitchYawFromRotationFCN(R_0)

    rollPitchYaw = rollPitchYawFromRotation(R_0);
end

== matlab function Visualization/Visualize Smoothing (orientation)/Rotation Error Right Foot/Rot error using roll-pitch-yaw ==
  data: R_0 input double; rollPitchYaw output double
function rollPitchYaw = rollPitchYawFromRotationFCN(R_0)

    rollPitchYaw = rollPitchYawFromRotation(R_0);
end

== matlab function Visualization/Visualize Smoothing (orientation)/Rotation Error Rot Task/Rot error using roll-pitch-yaw ==
  data: R_0 input double; rollPitchYaw output double
function rollPitchYaw = rollPitchYawFromRotationFCN(R_0)

    rollPitchYaw = rollPitchYawFromRotation(R_0);
end

== matlab function Robot State and References/State Machine/Compute Transformation Matrices/LFoot to base link transform/fromImuToHomogeousTransformFCN ==
  data: imu_H_link input double; imu_H_link_0 input double; link_H_base input double; inertial_0 input double; inertial input double; neck_pos input double; w_H_b output double; Config parameter double
function w_H_b = worldToBaseTransformWithIMUFCN(imu_H_link,imu_H_link_0,link_H_base,inertial_0,inertial,neck_pos,Config)

    w_H_b = worldToBaseTransformWithIMU(imu_H_link,imu_H_link_0,link_H_base,inertial_0,inertial,neck_pos,Config);

end
